simulink model "Aufgabe1_sim"  (R2023b)
settings: Solver=VariableStepAuto  StartTime=0.0  StopTime=20  RelTol=1e-3
values from neighbouring files (symbols this model uses):
  J = 4000e-7    (= 0.0004)    [Aufgabe1_param.m]
  K = 30e-3    (= 0.03)    [Aufgabe1_param.m]
  L = 120e-6    (= 0.00012)    [Aufgabe1_param.m]
  R = 6    [Aufgabe1_param.m]
settings Model: Creator=rouven  LastModifiedBy=rouven

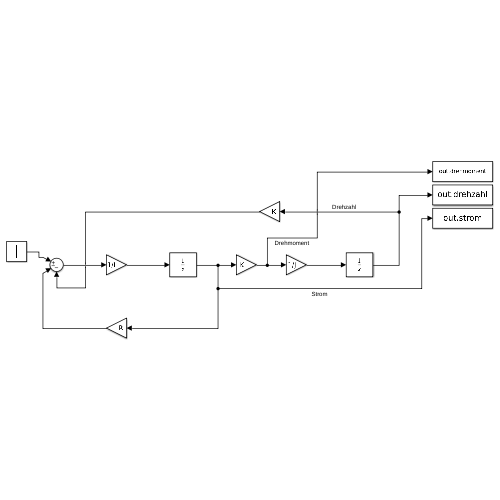
[thumbnail: Simulink's stored preview of the top-level diagram]
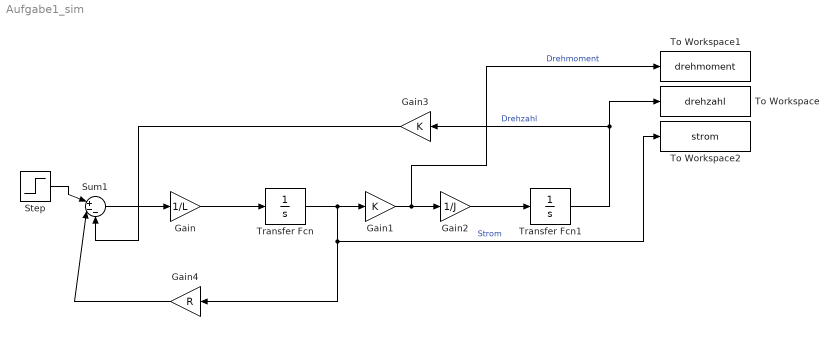
== system Aufgabe1_sim ==
  Gain : Gain  Gain=1/L
  Gain1 : Gain  Gain=K
  Gain2 : Gain  Gain=1/J
  Gain3 : Gain  Gain=K
  Gain4 : Gain  Gain=R
  Step : Step  After=10  SampleTime=0
  Sum1 : Sum  Inputs=|+--
  To Workspace : ToWorkspace  VariableName=drehzahl  SaveFormat=Structure With Time  SampleTime=-1
  To Workspace1 : ToWorkspace  VariableName=drehmoment  SaveFormat=Structure With Time  SampleTime=-1
  To Workspace2 : ToWorkspace  VariableName=strom  SaveFormat=Structure With Time  SampleTime=-1
  Transfer Fcn : TransferFcn  Denominator=[1 0]
  Transfer Fcn1 : TransferFcn  Denominator=[1 0]
  wires:
  Step/1 -> Sum1/1
  Sum1/1 -> Gain/1
  Gain/1 -> Transfer Fcn/1
  Gain1/1 -> To Workspace1/1, Gain2/1  "Drehmoment"
  Gain2/1 -> Transfer Fcn1/1
  Transfer Fcn1/1 -> To Workspace/1, Gain3/1  "Drehzahl"
  Transfer Fcn/1 -> To Workspace2/1, Gain4/1, Gain1/1  "Strom"
  Gain4/1 -> Sum1/2
  Gain3/1 -> Sum1/3
